simulink model "indicator_control_model"  (R2024b)
settings: Solver=FixedStepDiscrete  StartTime=0.0  StopTime=10.0  FixedStep=0.1  RelTol=1e-3
settings Model: Creator=siman  LastModifiedBy=siman
settings OptimizationCC: DefaultParameterBehavior=Inlined  EnhancedBackFolding=on  PassReuseOutputArgsAs=Individual arguments  ZeroExternalMemoryAtStartup=off  ZeroInternalMemoryAtStartup=off  OptimizeBlockOrder=speed  DifferentSizesBufferReuse=on  OptimizationCustomize=off  EfficientTunableParamExpr=on
settings DebuggingCC: ParameterTunabilityLossMsg=error  UnderSpecifiedDimensionMsg=error
settings SFSimCC: MATLABDynamicMemAlloc=off
settings RTWCC: Description=Embedded Coder  SystemTargetFile=ert.tlc  TemplateMakefile=ert_default_tmf
settings CodeAppCC: ForceParamTrailComments=on  IgnoreCustomStorageClasses=off  OperatorAnnotations=on  SimulinkDataObjDesc=on  SFDataObjDesc=on  InsertBlockDesc=on
settings ERTTargetCC: TargetLangStandard=C99 (ISO)  GenerateSampleERTMain=on  ERTCustomFileTemplate=example_file_process.tlc

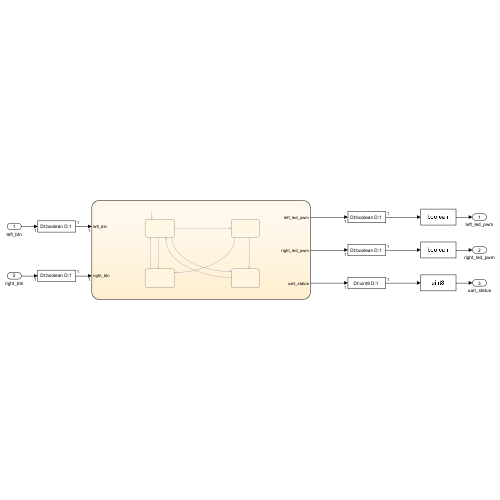
[thumbnail: Simulink's stored preview of the top-level diagram]
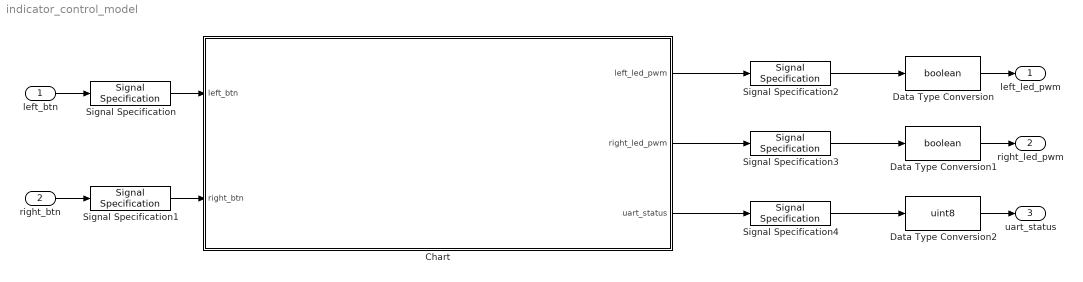
== system indicator_control_model ==
  left_btn : Inport
  right_btn : Inport  Port=2
  Chart : Stateflow chart  TreatAsAtomicUnit=on
  Data Type Conversion : DataTypeConversion  OutDataTypeStr=boolean  SaturateOnIntegerOverflow=off  RndMeth=Floor
  Data Type Conversion1 : DataTypeConversion  OutDataTypeStr=boolean  SaturateOnIntegerOverflow=off  RndMeth=Floor
  Data Type Conversion2 : DataTypeConversion  OutDataTypeStr=uint8  SaturateOnIntegerOverflow=off  RndMeth=Floor
  Signal Specification{,1..3} (4 alike) : SignalSpecification  OutDataTypeStr=boolean  Dimensions=1
  Signal Specification4 : SignalSpecification  OutDataTypeStr=uint8  Dimensions=1
  left_led_pwm : Outport
  right_led_pwm : Outport  Port=2
  uart_status : Outport  Port=3
  wires:
  Data Type Conversion/1 -> left_led_pwm/1
  Data Type Conversion1/1 -> right_led_pwm/1
  Data Type Conversion2/1 -> uart_status/1
  left_btn/1 -> Signal Specification/1
  Signal Specification/1 -> Chart/1(left_btn)
  right_btn/1 -> Signal Specification1/1
  Signal Specification1/1 -> Chart/2(right_btn)
  Chart/1(left_led_pwm) -> Signal Specification2/1
  Signal Specification2/1 -> Data Type Conversion/1
  Chart/2(right_led_pwm) -> Signal Specification3/1
  Signal Specification3/1 -> Data Type Conversion1/1
  Chart/3(uart_status) -> Signal Specification4/1
  Signal Specification4/1 -> Data Type Conversion2/1

== stateflow chart indicator_control_model/Chart ==
  state OFF
    entry:
    left_led_pwm = false;
    right_led_pwm = false;
    uart_status = 0; % this is fine because it's uint8
  state HAZARD
    entry:
    left_led_pwm = ~left_led_pwm;
    right_led_pwm = ~right_led_pwm;
  state LEFT_ON
    entry:
    left_led_pwm = ~left_led_pwm;  % fine
    right_led_pwm = false;
  state RIGHT_ON
    entry:
    right_led_pwm = ~right_led_pwm;
    left_led_pwm = false;
  (default) -> OFF
  OFF -> HAZARD [order 2] : [left_btn && right_btn]
  LEFT_ON -> OFF : [~left_btn && ~right_btn]
  OFF -> LEFT_ON [order 1] : [left_btn && ~right_btn]
  RIGHT_ON -> OFF : [~left_btn && ~right_btn]
  OFF -> RIGHT_ON [order 3] : [right_btn && ~left_btn]
  HAZARD -> LEFT_ON [order 1] : [left_btn && ~right_btn]
  HAZARD -> RIGHT_ON [order 2] : [right_btn && ~left_btn]
  data: left_btn input boolean size=1; right_btn input boolean size=1; left_led_pwm output boolean size=1; right_led_pwm output boolean size=1; uart_status output uint8 size=1
